simulink model "BallBeam_DigitalPID"  (R2016b)
settings: Solver=ode45  StartTime=0.0  StopTime=1000  RelTol=1e-3  EnableMultiTasking=on
InitFcn:
  | param
undefined symbols (not defined in the file or in its folder): ball_ctrl_state_int, drawBallSys, P
settings Model: Creator=beard  LastModifiedBy=Jacob
settings DataIOCC: LimitDataPoints=on  SaveFormat=Array  SignalLoggingSaveFormat=ModelDataLogs
settings OptimizationCC: ExpressionDepthLimit=2147483647  InitFltsAndDblsToZero=on  LifeSpan=inf
settings DebuggingCC: UnderspecifiedInitializationDetection=Classic  MergeDetectMultiDrivingBlocksExec=none  SolverPrmCheckMsg=warning  FcnCallInpInsideContextMsg=warning  StateNameClashWarn=warning  SFUnexpectedBacktrackingDiag=warning  SFNoUnconditionalDefaultTransitionDiag=warning  SFExecutionAtInitializationDiag=none
settings HardwareCC: ProdBitPerPointer=32  ProdBitPerSizeT=32  ProdBitPerPtrDiffT=32  ProdLargestAtomicFloat=None  ProdIntDivRoundTo=Undefined  ProdEndianess=Unspecified  ProdWordSize=32  ProdHWDeviceType=32-bit Generic
settings ModelReferenceCC: PropagateSignalLabelsOutOfModel=off
settings GRTTargetCC: TargetLangStandard=C89/C90 (ANSI)  GeneratePreprocessorConditionals=Disable all  CombineOutputUpdateFcns=off  GRTInterface=on
settings ConfigComp: CovMetricSettings=dw  CovHtmlReporting=on  CovSaveCumulativeToWorkspaceVar=on  CovSaveSingleToWorkspaceVar=on  CovExternalEMLEnable=off

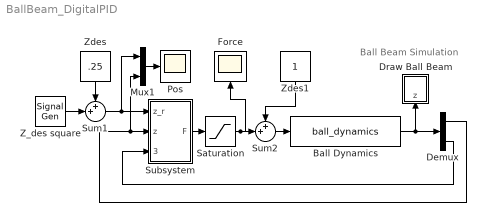
== system BallBeam_DigitalPID ==
  note: Ball Beam Simulation
  Ball Dynamics : S-Function  FunctionName=ball_dynamics  Parameters=P  SFunctionDeploymentMode=off  EnableBusSupport=off
  Demux : Demux  Outputs=2
  Draw Ball Beam : Subsystem
  Force : Scope
  Mux1 : Mux  Inputs=2
  Pos : Scope
  Saturation : Saturate  UpperLimit=25  LowerLimit=0
  Subsystem : Subsystem
  Sum1 : Sum  Inputs=++|
  Sum2 : Sum  Inputs=++|
  Z_des square : SignalGenerator  WaveForm=square  Amplitude=.15  Frequency=.5  Units=rad/sec
  Zdes : Constant  Value=.25
  Zdes1 : Constant
  wires:
  Ball Dynamics/1 -> Demux/1, Draw Ball Beam/1(z)
  Zdes/1 -> Sum1/1
  Z_des square/1 -> Sum1/2
  Mux1/1 -> Pos/1
  Subsystem/1(F) -> Saturation/1
  Sum1/1 -> Mux1/1, Subsystem/1(z_r)
  Demux/1 -> Mux1/2, Subsystem/2(z)
  Demux/2 -> Subsystem/3(theta)
  Saturation/1 -> Force/1, Sum2/2
  Zdes1/1 -> Sum2/1
  Sum2/1 -> Ball Dynamics/1

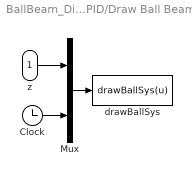
== system BallBeam_DigitalPID/Draw Ball Beam ==
  z : Inport
  Clock : Clock
  Mux : Mux  Inputs=2
  drawBallSys : MATLABFcn  MATLABFcn=drawBallSys(u)  OutputDimensions=0  SampleTime=.5
  wires:
  Mux/1 -> drawBallSys/1
  Clock/1 -> Mux/2
  z/1 -> Mux/1

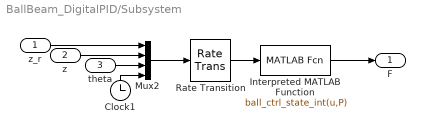
== system BallBeam_DigitalPID/Subsystem ==
  z_r : Inport
  z : Inport  Port=2
  theta : Inport  Port=3
  Clock1 : Clock
  Interpreted MATLAB Function : MATLABFcn  MATLABFcn=ball_ctrl_state_int(u,P)  OutputDimensions=1
  Mux2 : Mux
  Rate Transition : RateTransition  OutPortSampleTime=P.Ts
  F : Outport
  wires:
  Clock1/1 -> Mux2/4
  Mux2/1 -> Rate Transition/1
  Rate Transition/1 -> Interpreted MATLAB Function/1
  z_r/1 -> Mux2/1
  z/1 -> Mux2/2
  theta/1 -> Mux2/3
  Interpreted MATLAB Function/1 -> F/1
